simulink library "PreprocessingBlock"  (Simulink 10.1)
settings: Solver=ode45  StartTime=0.0  StopTime=10.0  RelTol=1e-3  EnableMultiTasking=on
libraries: simulink x9, dspsigattribs x4, Preprocessing x1, dspstat3 x1, SignalQuality x1
settings Model: Creator=g.tec medical engineering  ModifiedByFormat=g.tec  LastModifiedBy=g.tec

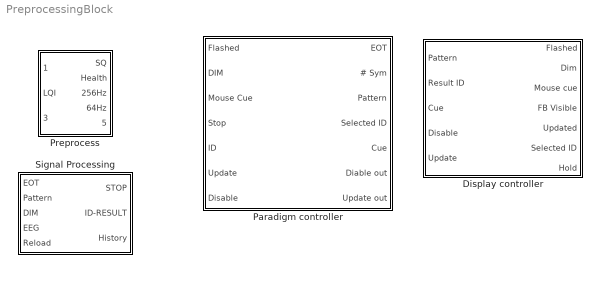
== system PreprocessingBlock ==
  Display controller : Subsystem  mask(Display controller){flashstyle=Faces, symbolopacity=Transparent, feedbackstyle=Highlighting, facetime=100, normaltime=70, feedbackduration=3, postfeedback=0.5, storagepath=XML_Paradigm\, maskfilename=, displayhost=127.0.0.1, displayhostport=11001, localport=11000, startdisplay=off}
      mask prompts: flashstyle "Flashing style"; symbolopacity "Symbol opacity"; feedbackstyle "Feedback style"; facetime "Face time [ms]"; normaltime "Normal time [ms]"; feedbackduration "Feedback duration [s]"; postfeedback "Post feedback break [s]"; storagepath "XML storage path"; maskfilename "XML mask file name"; displayhost "Display IP"; displayhostport "Display port"; localport "Controller port"; startdisplay "Auto start display (localhost only)"
      mask help:
      | Controls the output to the primary user interface based upon the
      | provided input patterns, the feedback information and the XML file
      | describing the symbols to be displayed and their order.
      mask init:
      | debug_Display_controller;
      settings: DeleteFcn=debug_Display_controller(true);
      mask Help:
      | Controls the output to the primary user interface based upon the
      | provided input patterns, the feedback information and the XML file
      | describing the symbols to be displayed and their order.
      | 
      | The following parameters can be used to define the style of the output and
      | on which system it should be displayed.
      | 
      | 
      | <b>Cursor style:</b> defines the style of the cursor used to step through
      | the individual symbols. The following values are avialable
      |     <i>Inverting</i> ...... inverts the colors of the symbols
      |     <i>Faces</i> .......... display images of well known people
      | 
      | <b>XML storage path</b> the pather where the mask description and all other
      | media are located. Must be equal to the path specified for the Interface unit
      | 
      | <b>XML mask file name</b> the name of the file describing the symbols to
      | be displayed.
      | 
      | <b>Display IP</b> the ip address of the computer connected to the user
      | display
      | 
      | <b>Display port</b> the port the display is receiving messages from the
      | controller.
      | 
      | <b>Controller port</b> the port the controller is receiving response messages
      | from the display
      | 
      | <b>Auto start dispaly (localhot only)</b> if set than the display application
      | is started if necessary. It will not be started wither whien this controll is
      | off or when <b>Display IP</b> is not set to localhost (127.0.0.1)
      mask TypeOptions flashstyle: Inverting | Faces
      mask TypeOptions symbolopacity: Transparent | Solid
      mask TypeOptions feedbackstyle: Fullscreen | Highlighting
      mask Display:
      | image(imread('soci.jpg'))
      | 
      | port_label('output', 1, 'Flashed')
      | port_label('output', 2, 'Dim')
      | port_label('output', 3, 'Mouse Cue')
      | port_label('output', 4, 'FB visible')
      | port_label('output', 5, 'Updated')
      | port_label('output', 7, 'Hold')
      | port_label('output', 6, 'Selected ID')
      | port_label('input', 1, 'Pattern')
      | port_label('input', 2, 'Result ID')
      | port_label('input', 3, 'Cue')
      | port_label('input', 4, 'Disable')
      | port_label('input', 5, 'Update')
  Paradigm controller : Subsystem  mask(Paradigm controler){opmode=Training, patterntype=Row/Column, maxpatternsize=11, screenfrequency=60}
      mask prompts: opmode "Mode"; patterntype "Pattern type"; maxpatternsize "Max pattern size"; screenfrequency "Refresh rate [Hz]"
      mask help: Controls the workflow of the P300 BCI
      mask init:
      | initializeParadigm
      mask TypeOptions opmode: Training | Copy spelling | Free spelling
      mask TypeOptions patterntype: Single | Row/Column | Random pattern
      mask Display:
      | image(imread('speller2.png'))
      | port_label('input',1,'Flashed')
      | port_label('input',2,'DIM')
      | port_label('input',3,'Mouse Cue')
      | port_label('input',4,'Stop')
      | port_label('input',5,'ID')
      | port_label('input',6,'Update')
      | port_label('input',7,'Disable')
      | port_label('output',1,'EOT')
      | port_label('output',2,'SYM')
      | port_label('output',3,'Pattern')
      | port_label('output',4,'Selected ID')
      | port_label('output',5,'Cue')
      | port_label('output',6,'Disable out')
      | port_label('output',7,'Update out')
  Preprocess : Subsystem  mask(Preprocessing){adjustsignalquality=off, adjustfiltersettings=off, numinvalid=8, batterylevels=[30,5], linkquality=[ 50 6], samplingfactor=4}
      mask prompts: adjustsignalquality "Adjust signal quality settings"; adjustfiltersettings "Adjust input filter settings"; numinvalid "Stop if more than # channels are invalid"; batterylevels "Batterly levels [%] (Warn, Off)"; linkquality "Link Quality [%] ( Warn, Lost)"; samplingfactor "Sampling factor"
      mask help:
      | Applys all necessary preprocessing stepts to the in comming raw data
      | This includes downsampling to 64 Hz, checking the quality and reliability of the signals and applying any necessary filtering step
      mask init:
      | hh = get(0,'ShowHiddenHandles');    
      | try
      |     close_system([[bdroot(gcb),'/Preprocess'],'/g.SQcheck'])
      |     set(0,'ShowHiddenHandles','on');
      |     sqck = findobj('name','Online Signal Quality Check');    
      |     set(0,'ShowHiddenHandles',hh);
      |     close(sqck);
      | catch
      |     set(0,'ShowHiddenHandles',hh);
      | end
      | try
      |     close_system([[bdroot(gcb),'/Preprocess'],'/Bandpass Butterworth Filter'])
      | catch
      | end
      | 
      | set_param([[bdroot(gcb),'/Preprocess'],'/Num invalid channels'],'const',numinvalid)
      | set_param([[bdroot(gcb),'/Preprocess'],'/Downsample'],'N',samplingfactor)
      | if length(batterylevels) < 2 || batterylevels(2) >= 100 || batterylevels(2) <= 0
      |     batterylevels(2) = 5;
      | end
      | if batterylevels(1) < batterylevels(2) 
      |     batterylevels(1) = batterylevels(2);
      | end
      | if length(linkquality) < 2 || linkquality(2) >= 100 || linkquality(2) <= 0 
      |     linkquality(2) = 10;
      | end
      | if linkquality(1) < linkquality(2)
      |     linkquality(1) = linkquality(2);
      | end
      | set_param([[bdroot(gcb),'/Preprocess'],'/Off Lim'],'const',sprintf('[%.1f,%.1f]',linkquality(2),batterylevels(2)));
      | set_param([[bdroot(gcb),'/Preprocess'],'/Warn Lim'],'const',sprintf('[%.1f,%.1f]',linkquality(1),batterylevels(1)));
      mask Callback adjustsignalquality: openSQcheck
      mask Callback adjustfiltersettings: openFilterSettings
      mask Display:
      | port_label('Input',1,'Raw EEG')
      | port_label('Input',2,'LQI')
      | port_label('Input',3,'Batt')
      | port_label('Output',1,'SQ')
      | port_label('Output',2,'Health')
      | 
      | try
      |     sfreq = 1/str2num(get(get_param(bdroot(gcb),'Handle'),'FixedStep'));
      |     if ~exist('sfreq','var') || size(sfreq,1) ~= 1 || size(sfreq,2) ~= 1 || length(size(sfreq))>2
      |         sreq = 256;
      |     end
      | catch ME
      |     sfreq = 256;
      | 
      | end
      | ds = sfreq/str2num(get_param(gcb,'samplingfactor'));
      | port_label('Output',3,sprintf('%.0f Hz',sfreq));
      | port_label('Output',4,sprintf('%.1f Hz',ds));
      | port_label('Output',5,'Signal bad');
  Signal Processing : Subsystem  AncestorBlock=PreprocessingBlock/Signal Processing  mask(P300 Signal Processing){windTime=800, runmax=15, method=Linear Discriminant Analysis, evaluationmethod=Fixed number of flashes, canselect=0.35, classifierfile=Subject_1_training_31_03_2021_08_35_44_0000_LDA.mat, sharedwith=1}
      mask prompts: windTime "Buffer length [ms]"; runmax "Number of flashes:"; method "Classification method:"; evaluationmethod "Evaluation method:"; canselect "Global residual error probability [%]"; classifierfile "Clasifier file"; sharedwith "Shared With"
      mask help:
      | The block buffers EEG data for each ID-Flash obtained. As soon as M
      | (Number of flashes) characters of each ID are obtained, or a decision may
      | be taken on the symbol selected by the user when one of the statistical
      | evaluation methods  is selceted, a STOP command is sent and the maximum
      | P300 is calculated and applied on output ID.
      mask init:
      | try
      | clobj = {};
      | try
      |     classifierhandle = matfile(classifierfile);
      |     classifierhandle = classifierhandle.P300Classifier;
      |     totalclasses = classifierhandle.numClasses;
      |     if totalclasses < 2
      |         totalclasses = 2;
      |     end
      |     set_param(gcb,'method',classifierhandle.methodName);
      | catch mee
      |     disp(getReport(mee))
      |     disp('safe')
      |     totalclasses = 2;
      | end
      | if ~isempty(clobj)
      |     clear(clobj{:});
      | end
      | catch me
      |     disp(getReport(me));
      |     disp('bad')
      | end
      mask Help:
      | P300 Signal Processing block. The block buffers EEG data for each ID-Flash
      | obtained. As soon as M (Number of flashes) characters of each ID are
      | obtained, or a decision may be taken on the symbol selected by the user
      | when one of the statistical approaches is selceted, a STOP command is sent
      | and the maximum P300 is calculated and applied on output ID.<br>
      | 
      | <b>Buffer length [ms]</b> - enter the EEG data buffer size <br><br>
      | 
      | <b>Number of flashes</b> - enter the number each character should flash up <br><br>
      | 
      | <b>Classification method</b> - names the method used for classifying the data
      |                            corresponding to each individual flash pattern.
      |                            The used method is defined by the classifier loaed
      |                            For example the following are supported<br>
      |    LDA ... Linear discriminant analysis (default) <br>
      |    SVM ... Support vector machines <br><br>
      | 
      | <b>Evaluation method</b> - Approach used to identify the symbol selected by
      |                            the users <br>
      |     <i>Fixed number of flashes</i>
      |         No output will be generated before not all symbols/rows/columns have
      |         flashed at leased <b>Number of flashes times</b><br>
      | 
      |     <i>Global P statistics</i>
      |         After each flash cycle the global scores for each symbol are updated.
      |         If the residual error of at least one symbol drops below the value
      |         specified for the <b>Global residual error probability</b> parameter,
      |         the flashing stops and the ID is set to the corresponding symbol
      |         identifier<br>
      | 
      |    <i>Fixed number of flashes with global P-statistics</i>
      |         A combination of the <i>Fixed number of flasehs</i> and the
      |         <i>Global P-statistics</i> modes.
      | 
      | <b>Global residual error probability [%]</b> - The residual error probability
      |     limit which is used by the <i>Global p statistics</i> and the
      |     <i>Per run P statistics</i> mode to determine whether a decision about
      |     the chosen symbol may be taken or not.
      | 
      |     <i>NOTE:</i> if set to empty value than the following polynome will be
      |                  used to compute an appropriate value<br><br>
      |     <center> ci = -0.002748869222306 * nfl^3  + 0.102514650781359 * nfl^2 -1.290670937088071 * nfl + 5.858716739649105</center>
      | 
      | <b>Clasifier file</b> - The name of a valid P300classifier file.
      mask TypeOptions evaluationmethod: Fixed number of flashes | Global P statistics | Fixed number of flashes with global P-statistics
      mask Display:
      | image(imread('p300.png'))
      | port_label('output', 1, 'STOP')
      | port_label('output', 2, 'ID')
      | port_label('output', 3, 'History')
      | port_label('input', 4, 'EEG')
      | port_label('input', 3, 'DIM')
      | port_label('input', 1, 'EOT')
      | port_label('input', 2, 'Pattern')
      | port_label('input', 5, 'Reload')

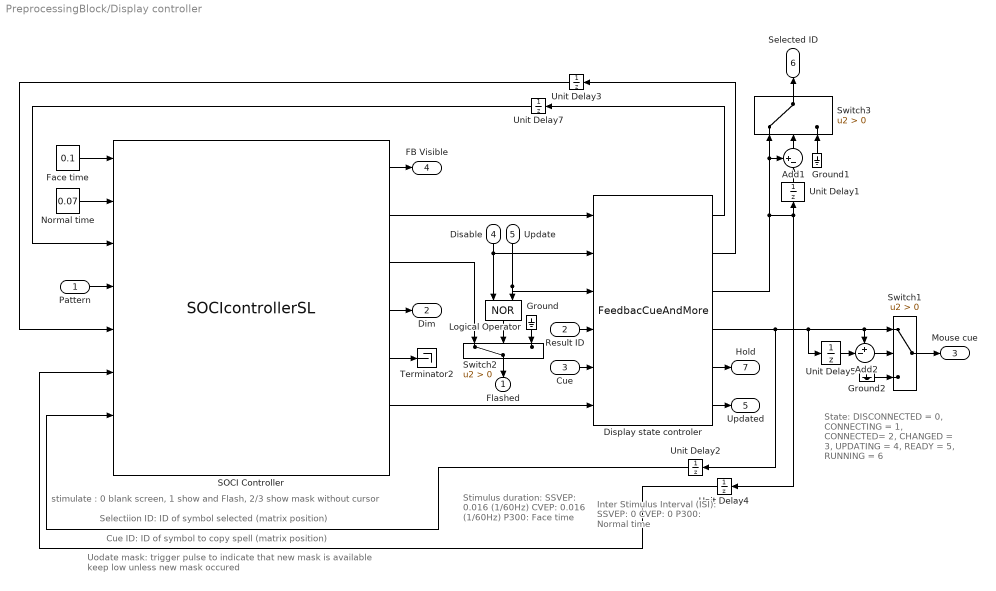
== system PreprocessingBlock/Display controller ==
  note: Uodate mask: trigger pulse to indicate that new mask is available
      |  keep low unless new mask occured
  note: Cue ID: ID of symbol to copy spell (matrix position)
  note: Selectiion ID: ID of symbol selected (matrix position)
  note: Inter Stimulus Interval (ISI):
      | SSVEP: 0
      | CVEP: 0
      | P300: Normal time
  note: Stimulus duration:
      |  SSVEP: 0.016 (1/60Hz)
      | CVEP: 0.016 (1/60Hz)
      |  P300: Face time
  note: State:
      | DISCONNECTED = 0,
      |  CONNECTING = 1,
      |  CONNECTED= 2,
      |  CHANGED = 3,
      | UPDATING = 4,
      | READY = 5,
      |  RUNNING = 6
  note: stimulate : 0 blank screen, 1 show and Flash, 2/3 show mask without cursor
  Pattern : Inport
  Result ID : Inport  Port=2
  Cue : Inport  Port=3
  Disable : Inport  Port=4
  Update : Inport  Port=5
  Add1 : Sum  Inputs=+-|
  Add2 : Sum  Inputs=+-|
  Display state controler : M-S-Function  FunctionName=FeedbacCueAndMore  Parameters=DelayLength,PostFeedback  mask{DelayLength=3, PostFeedback=0.5}
      mask prompts: DelayLength "Feedback & Cue delay [s]"; PostFeedback "Post feedback break [s]"
      mask Display:
      | port_label('input',2,'Disable')
      | port_label('input',3,'Update')
      | port_label('input',1,'Mouse trigger')
      | port_label('input',4,'Result ID')
      | port_label('input',5,'Cue')
      | port_label('input',6,'State')
      | port_label('output',1,'Stimulate')
      | port_label('output',2,'Update mask')
      | port_label('output',3,'Feedback')
      | port_label('output',4,'Show cue')
      | port_label('output',5,'Hold')
      | port_label('output',6,'Updated')
  Face time : Constant  Value=0.1
  Ground : Ground
  Ground1 : Ground
  Ground2 : Ground
  Logical Operator : Logic  Operator=NOR  AllPortsSameDT=off  OutDataTypeStr='double'
  Normal time : Constant  Value=0.07
  SOCI Controller : S-Function  FunctionName=SOCIcontrollerSL  Parameters=flashMode, opacityMode, feedbackMode, stimulusTransmission, maskFilename, mediaPath, maxRows, maxColumns, displayIP, displayPort, controllerPort, autostartDisplay, patternStyle, presentationOrder, maskStyle  SFunctionDeploymentMode=off  EnableBusSupport=off  mask{flashMode=Faces, opacityMode=Transparent, feedbackMode=Highlighting, stimulusTransmission=Queue stimulation pattern in FIFO buffer, patternStyle=Index vector, maskFilename=XML_Initialisation_Tactile_2Stim.xml, mediaPath=\SociMediaFiles\, maskStyle=Matrix, maxRows=0, maxColumns=0, presentationOrder=Deterministic, displayIP=127.0.0.1, displayPort=11001, controllerPort=11000, autostartDisplay=on}
      mask prompts: flashMode "Flash mode"; opacityMode "Opacity"; feedbackMode "Feedback"; stimulusTransmission "Stimulus transmission"; patternStyle "Pattern style"; maskFilename "XML mask file"; mediaPath "Media path"; maskStyle "XML mask style"; maxRows "Max rows"; maxColumns "Max columns"; presentationOrder "Icon group presenation"; displayIP "Display IP"; displayPort "Display Port"; controllerPort "Controller Port"; autostartDisplay "Autostart display (localhost only)"
      mask TypeOptions flashMode: Highlighting | Inverting | Faces
      mask TypeOptions opacityMode: Transparent | Solid
      mask TypeOptions feedbackMode: Fullscreen | Highlighting | Frame
      mask TypeOptions stimulusTransmission: Stream stimulation pattern without buffering | Queue stimulation pattern in FIFO buffer
      mask TypeOptions patternStyle: Binary vector | Index vector
      mask TypeOptions maskStyle: Matrix | Collection
      mask TypeOptions presentationOrder: Deterministic | Randomized
      mask DialogControl Control1 Prompt: Scaling of the mask (enter 0 for autoscaling)
      mask Display:
      | image('soci.jpg')
      | port_label('output', 1, 'Feedback trigger')
      | port_label('output', 2, 'Mouse trigger')
      | port_label('output', 3, 'Pattern trigger')
      | port_label('output', 4, 'Mask definition')
      | port_label('output', 5, 'Display rate')
      | port_label('output', 6, 'State')
      | 
      | port_label('input', 1, 'Stimulus duration (s) (FIFO only)')
      | port_label('input', 2, 'ISI (s) (FIFO only)')
      | port_label('input', 3, 'Stimulate')
      | port_label('input', 4, 'Stimulation pattern')
      | port_label('input', 5, 'Update mask')
      | port_label('input', 6, 'Selection ID')
      | port_label('input', 7, 'Cue ID')
  Switch1 : Switch  Criteria=u2 > Threshold
  Switch2 : Switch  Criteria=u2 > Threshold
  Switch3 : Switch  Criteria=u2 > Threshold
  Terminator2 : Terminator
  Unit Delay{1..5,7} (6 alike) : UnitDelay  SampleTime=-1  HasFrameUpgradeWarning=on
  Flashed : Outport
  Dim : Outport  Port=2
  Mouse cue : Outport  Port=3
  FB Visible : Outport  Port=4
  Updated : Outport  Port=5
  Selected ID : Outport  Port=6
  Hold : Outport  Port=7
  wires:
  SOCI Controller/4 -> Dim/1
  Pattern/1 -> SOCI Controller/4
  SOCI Controller/1 -> FB Visible/1
  SOCI Controller/5 -> Terminator2/1
  Unit Delay1/1 -> Add1/2
  Switch3/1 -> Selected ID/1
  Add1/1 -> Switch3/2
  Display state controler/2 -> Unit Delay3/1
  Normal time/1 -> SOCI Controller/2
  Face time/1 -> SOCI Controller/1
  Ground1/1 -> Switch3/3
  Display state controler/6 -> Updated/1
  Display state controler/5 -> Hold/1
  Display state controler/1 -> Unit Delay7/1
  SOCI Controller/2 -> Display state controler/1
  Switch1/1 -> Mouse cue/1
  Result ID/1 -> Display state controler/4
  Cue/1 -> Display state controler/5
  SOCI Controller/6 -> Display state controler/6
  Unit Delay7/1 -> SOCI Controller/3
  Unit Delay3/1 -> SOCI Controller/5
  Display state controler/4 -> Unit Delay2/1, Add2/1, Switch1/1, Unit Delay5/1
  Display state controler/3 -> Add1/1, Switch3/1, Unit Delay4/1, Unit Delay1/1
  Unit Delay2/1 -> SOCI Controller/7
  Unit Delay4/1 -> SOCI Controller/6
  Logical Operator/1 -> Switch2/2
  Ground/1 -> Switch2/3
  Disable/1 -> Logical Operator/1, Display state controler/2
  Update/1 -> Display state controler/3, Logical Operator/2
  Ground2/1 -> Switch1/3
  SOCI Controller/3 -> Switch2/1
  Switch2/1 -> Flashed/1
  Add2/1 -> Switch1/2
  Unit Delay5/1 -> Add2/2

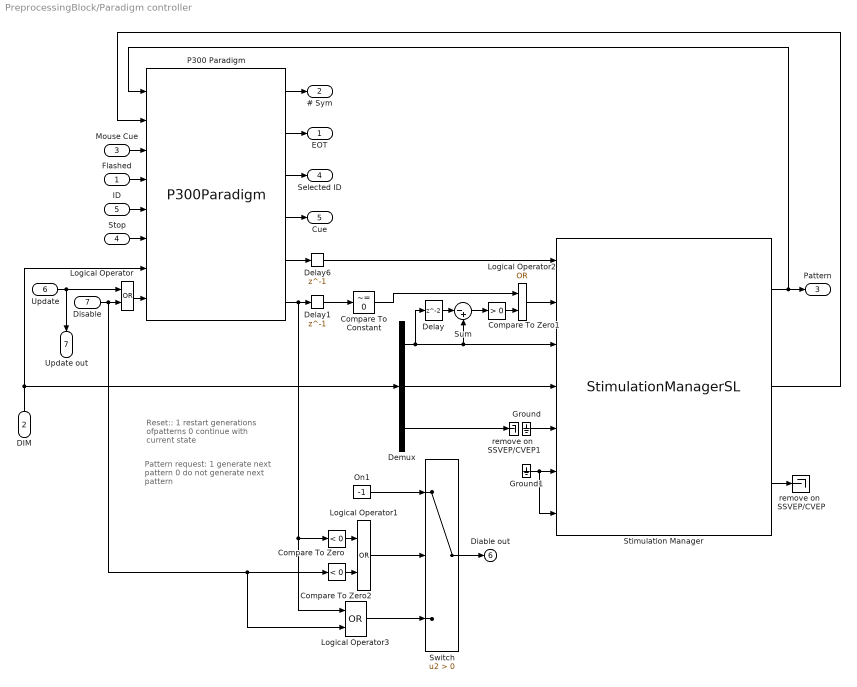
== system PreprocessingBlock/Paradigm controller ==
  note: Pattern request:
      | 1 generate  next pattern
      | 0 do not generate next pattern
  note: Reset::
      | 1 restart generations ofpatterns
      | 0 continue with current state
  Flashed : Inport
  DIM : Inport  Port=2
  "Mouse Cue\t" : Inport  Port=3
  Stop : Inport  Port=4
  ID : Inport  Port=5
  Update : Inport  Port=6
  Disable : Inport  Port=7
  Compare To Constant : simulink/Logic and Bit Operations/Compare To Constant  relop=~=  const=0  OutDataTypeStr=boolean
  Compare To Zero : simulink/Logic and Bit Operations/Compare To Zero  relop=<  OutDataTypeStr=boolean
  Compare To Zero1 : simulink/Logic and Bit Operations/Compare To Zero  relop=>  OutDataTypeStr=boolean
  Compare To Zero2 : simulink/Logic and Bit Operations/Compare To Zero  relop=<  OutDataTypeStr=boolean
  Delay : Delay
  Delay1 : Delay  DelayLength=1  InitialCondition=0
  Delay6 : Delay  DelayLength=1  InitialCondition=0
  Demux : Demux  Outputs=3
  Ground : Ground
  Ground1 : Ground
  Logical Operator{,1..3} (4 alike) : Logic  Operator=OR  AllPortsSameDT=off  OutDataTypeStr='double'
  On1 : Constant  Value=-1
  P300 Paradigm : M-S-Function  FunctionName=P300Paradigm  Parameters=patternsize,operationmode,expectfirstpatternlatest  mask{operationmode=Training, patternsize=11, expectfirstpatternlatest=1/60}
      mask prompts: operationmode "Mode"; patternsize "Pattern size"; expectfirstpatternlatest "Expect first pattern latest"
      mask TypeOptions operationmode: Training | Copy spelling | Free spelling
      mask Display:
      | port_label('input',1,'Pattern')
      | port_label('input',2,'Trial end')
      | port_label('input',3,'Mouse cue')
      | port_label('input',4,'Flashed')
      | port_label('input',5,'ID')
      | port_label('input',6,'Stop')
      | port_label('input',8,'Disable')
      | port_label('input',7,'DIM')
      | port_label('output',1,'# Symbols')
      | port_label('output',2,'EOT')
      | port_label('output',3,'Selected ID')
      | port_label('output',4,'Cue')
      | port_label('output',5,'Request')
      | port_label('output',6,'Reset')
  Stimulation Manager : S-Function  FunctionName=StimulationManagerSL  Parameters=patternType, patternSize, holdPattern, outputType, holdSamples, updateRate  SFunctionDeploymentMode=off  EnableBusSupport=off  mask{patternType=Row/Column, patternSize=11, holdPattern=off, holdSamples=1, outputType=Index vector, updateRate=60}
      mask prompts: patternType "Pattern type"; patternSize "Maximum pattern size"; holdPattern "Hold pattern until next request"; holdSamples "Minimum hold duration (in samples)"; outputType "Output type"; updateRate "Update rate of the stimulator (Hz)"
      mask TypeOptions patternType: Single | Row/Column | Random pattern | Constant frequency stimulation | Code based stimulation
      mask TypeOptions outputType: Binary vector | Index vector
      mask Display:
      | image('sequencer.jpg')
      | port_label('output', 1, 'Current pattern')
      | port_label('output', 2, 'Trial end')
      | port_label('output', 3, 'Phase shift (code based only)')
      | port_label('input', 1, 'Pattern request')
      | port_label('input', 2, 'Reset')
      | port_label('input', 3, '#rows')
      | port_label('input', 4, '#cols')
      | port_label('input', 5, 'Add pattern')
      | port_label('input', 6, 'Frequencies (constant frequency only)')
      | port_label('input', 7, 'Phase shift (code based only)')
  Sum : Sum  Inputs=|-+
  Switch : Switch  Criteria=u2 > Threshold
  remove on  SSVEP/CVEP : Terminator
  remove on  SSVEP/CVEP1 : Terminator
  EOT : Outport
  # Sym : Outport  Port=2
  Pattern : Outport  Port=3
  Selected ID : Outport  Port=4
  Cue : Outport  Port=5
  Diable out : Outport  Port=6
  Update out : Outport  Port=7
  wires:
  Stimulation Manager/2 -> P300 Paradigm/2
  Stimulation Manager/3 -> remove on  SSVEP/CVEP/1
  Demux/1 -> Delay/1, Sum/2, Stimulation Manager/3
  Demux/2 -> Stimulation Manager/4
  Ground/1 -> Stimulation Manager/5
  Ground1/1 -> Stimulation Manager/7, Stimulation Manager/6
  Update/1 -> Logical Operator/1, Update out/1
  Demux/3 -> remove on  SSVEP/CVEP1/1
  Flashed/1 -> P300 Paradigm/4
  Stop/1 -> P300 Paradigm/6
  ID/1 -> P300 Paradigm/5
  "Mouse Cue\t"/1 -> P300 Paradigm/3
  DIM/1 -> P300 Paradigm/7, Demux/1
  Stimulation Manager/1 -> P300 Paradigm/1, Pattern/1
  Delay6/1 -> Stimulation Manager/1
  P300 Paradigm/6 -> Logical Operator3/1, Compare To Zero/1, Delay1/1
  P300 Paradigm/5 -> Delay6/1
  P300 Paradigm/4 -> Cue/1
  P300 Paradigm/3 -> Selected ID/1
  P300 Paradigm/2 -> EOT/1
  P300 Paradigm/1 -> # Sym/1
  Delay1/1 -> Compare To Constant/1
  Compare To Constant/1 -> Logical Operator2/1
  Logical Operator2/1 -> Stimulation Manager/2
  Logical Operator/1 -> P300 Paradigm/8
  Switch/1 -> Diable out/1
  Logical Operator1/1 -> Switch/2
  On1/1 -> Switch/1
  Logical Operator3/1 -> Switch/3
  Compare To Zero/1 -> Logical Operator1/1
  Compare To Zero2/1 -> Logical Operator1/2
  Disable/1 -> Logical Operator3/2, Compare To Zero2/1, Logical Operator/2
  Compare To Zero1/1 -> Logical Operator2/2
  Delay/1 -> Sum/1
  Sum/1 -> Compare To Zero1/1

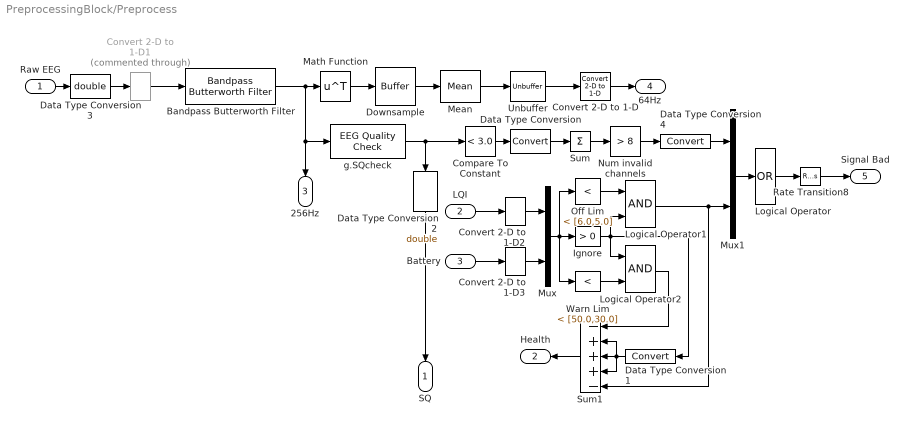
== system PreprocessingBlock/Preprocess ==
  Raw EEG : Inport
  LQI : Inport  Port=2
  Battery : Inport  Port=3
  Bandpass Butterworth Filter : Preprocessing/Bandpass Butterworth Filter  LPOrder=5  UpperFreq=30  HPOrder=5  LowerFreq=0.1  SampFreq=256
      settings: SourceProductName=g.HIsys
  Compare To Constant : simulink/Logic and Bit Operations/Compare To Constant  relop=<  const=3.0  OutDataTypeStr=boolean
  Convert 2-D to 1-D : dspsigattribs/Convert 2-D to 1-D
      settings: SourceProductBaseCode=DS
  Convert 2-D to 1-D1 : dspsigattribs/Convert 2-D to 1-D  Commented=through
      settings: SourceProductBaseCode=DS
  Convert 2-D to 1-D2 : dspsigattribs/Convert 2-D to 1-D
      settings: SourceProductBaseCode=DS
  Convert 2-D to 1-D3 : dspsigattribs/Convert 2-D to 1-D
      settings: SourceProductBaseCode=DS
  Data Type Conversion : DataTypeConversion
  Data Type Conversion1 : DataTypeConversion
  Data Type Conversion2 : DataTypeConversion  OutDataTypeStr=double
  Data Type Conversion3 : DataTypeConversion  OutDataTypeStr=double
  Data Type Conversion4 : DataTypeConversion
  Downsample : Buffer  N=4
  Ignore : simulink/Logic and Bit Operations/Compare To Constant  relop=>  const=0  OutDataTypeStr=boolean
  Logical Operator : Logic  Operator=OR  Inputs=1  AllPortsSameDT=off  OutDataTypeStr='double'
  Logical Operator1 : Logic  AllPortsSameDT=off  OutDataTypeStr='double'
  Logical Operator2 : Logic  AllPortsSameDT=off  OutDataTypeStr='double'
  Math Function : Math  Operator=transpose  SignedPower=on  SaturateOnIntegerOverflow=on
  Mean : dspstat3/Mean  run=off  InputProcessing=Columns as channels (frame based)  reset_popup=None  directionMode=Each column  dimension=1  roiEnable=off  roiType=Rectangles  roiPortion=Entire ROI  roiOutput=Individual statistics for each ROI  roiFlag=off  roundingMode=Floor  overflowMode=off  outputDataTypeStr=Inherit: Same as accumulator  outputMin=[]  outputMax=[]  outputLastDataTypeStr=Inherit: Same as accumulator
  Mux : Mux  Inputs=2
  Mux1 : Mux  Inputs=2
  Num invalid channels : simulink/Logic and Bit Operations/Compare To Constant  relop=>  const=8  OutDataTypeStr=boolean
  Off Lim : simulink/Logic and Bit Operations/Compare To Constant  relop=<  const=[6.0,5.0]  OutDataTypeStr=boolean
  Rate Transition8 : RateTransition
  Sum : Sum  Inputs=+
  Sum1 : Sum  Inputs=-+++-
  Unbuffer : Unbuffer
  Warn Lim : simulink/Logic and Bit Operations/Compare To Constant  relop=<  const=[50.0,30.0]  OutDataTypeStr=boolean
  g.SQcheck : SignalQuality/EEG Quality Check  stddev_enable=on  stddev_upper_limit=25  stddev_lower_limit=2.5  stddev_window=1000  stddev_unit=1  level_enable=off  level_upper_limit=100  level_lower_limit=10  level_window=500  level_unit=1
      settings: SourceProductName=g.HIsys
  SQ : Outport
  Health : Outport  Port=2
  256Hz : Outport  Port=3
  64Hz : Outport  Port=4
  Signal Bad : Outport  Port=5
  wires:
  Raw EEG/1 -> Data Type Conversion3/1
  Downsample/1 -> Mean/1
  Mean/1 -> Unbuffer/1
  Unbuffer/1 -> Convert 2-D to 1-D/1
  Convert 2-D to 1-D/1 -> 64Hz/1
  Compare To Constant/1 -> Data Type Conversion/1
  Data Type Conversion/1 -> Sum/1
  Sum/1 -> Num invalid channels/1
  Num invalid channels/1 -> Data Type Conversion4/1
  Logical Operator/1 -> Rate Transition8/1
  Rate Transition8/1 -> Signal Bad/1
  g.SQcheck/1 -> Data Type Conversion2/1, Compare To Constant/1
  Data Type Conversion2/1 -> SQ/1
  Data Type Conversion3/1 -> Convert 2-D to 1-D1/1
  Convert 2-D to 1-D1/1 -> Bandpass Butterworth Filter/1
  Battery/1 -> Convert 2-D to 1-D3/1
  LQI/1 -> Convert 2-D to 1-D2/1
  Off Lim/1 -> Logical Operator1/1
  Warn Lim/1 -> Logical Operator2/2
  Convert 2-D to 1-D2/1 -> Mux/1
  Convert 2-D to 1-D3/1 -> Mux/2
  Mux/1 -> Off Lim/1, Warn Lim/1, Ignore/1
  Mux1/1 -> Logical Operator/1
  Ignore/1 -> Data Type Conversion1/1, Logical Operator1/2, Logical Operator2/1
  Logical Operator2/1 -> Sum1/1
  Logical Operator1/1 -> Sum1/5, Mux1/2
  Data Type Conversion1/1 -> Sum1/3, Sum1/2, Sum1/4
  Sum1/1 -> Health/1
  Data Type Conversion4/1 -> Mux1/1
  Bandpass Butterworth Filter/1 -> Math Function/1, 256Hz/1, g.SQcheck/1
  Math Function/1 -> Downsample/1

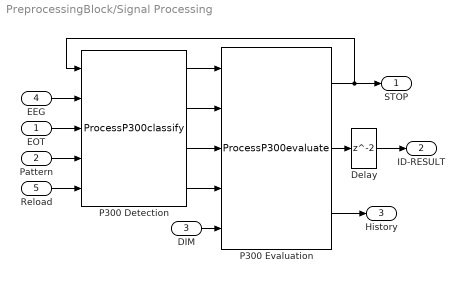
== system PreprocessingBlock/Signal Processing ==
  EOT : Inport
  Pattern : Inport  Port=2
  DIM : Inport  Port=3
  EEG : Inport  Port=4
  Reload : Inport  Port=5
  Delay : Delay  InitialCondition=0  InputProcessing=Columns as channels (frame based)
  P300 Detection : M-S-Function  FunctionName=ProcessP300classify  Parameters=windTime, totalclasses,classifierfile
      mask Display:
      | port_label('input',1,'Reset')
      | port_label('input',2,'EEG')
      | port_label('input',3,'EOT i')
      | port_label('input',4,'Pattern i')
      | port_label('input',5,'Reload')
      | port_label('Output',1,'Distance')
      | port_label('Output',2,'p-value')
      | port_label('Output',3,'Pattern o')
      | port_label('Output',4,'EOT o')
  P300 Evaluation : M-S-Function  FunctionName=ProcessP300evaluate  Parameters=runmax,evaluationmethod,canselect,0
      mask Display:
      | port_label('input',1,'Distance')
      | port_label('input',2,'p-Value')
      | port_label('input',3,'Pattern')
      | port_label('input',4,'EOT')
      | port_label('input',5,'DIM')
      | port_label('Output',1,'Stop')
      | port_label('Output',2,'ID-result')
      | port_label('Output',3,'History')
  STOP : Outport
  ID-RESULT : Outport  Port=2
  History : Outport  Port=3
  wires:
  P300 Detection/4 -> P300 Evaluation/4
  P300 Detection/3 -> P300 Evaluation/3
  Delay/1 -> ID-RESULT/1
  P300 Evaluation/1 -> STOP/1, P300 Detection/1
  EOT/1 -> P300 Detection/3
  Reload/1 -> P300 Detection/5
  P300 Evaluation/3 -> History/1
  P300 Detection/2 -> P300 Evaluation/2
  P300 Detection/1 -> P300 Evaluation/1
  Pattern/1 -> P300 Detection/4
  EEG/1 -> P300 Detection/2
  DIM/1 -> P300 Evaluation/5
  P300 Evaluation/2 -> Delay/1
